simulink model "ELECTRIC_RC_AIRCRAFT_backup_2"  (R2025b)
settings: Solver=VariableStepAuto  StartTime=0.0  StopTime=10000  RelTol=1e-3
values from neighbouring files (symbols this model uses):
  g = 9.81    [ELECTRIC_RC_AIRCRAFT.m]
  m = 1.83    [ELECTRIC_RC_AIRCRAFT.m]
libraries: aerolibadyn x1, aerolibatmos2 x1, aerolibasang x1, aerolibbdyn x1, aerolibactuator x1, slpidlib x1, aerolibpropulsion2 x1
settings Model: PacingRate=10  Creator=papar  LastModifiedBy=papar

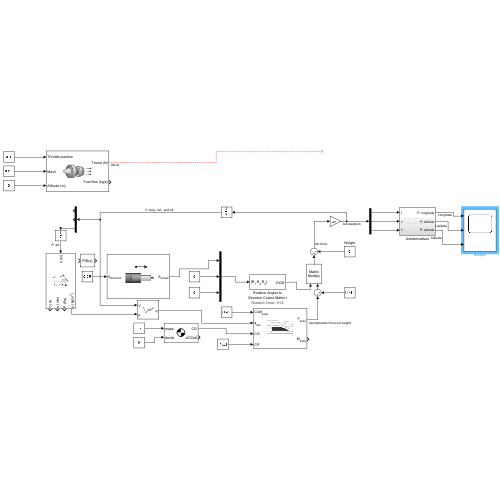
[thumbnail: Simulink's stored preview of the top-level diagram]
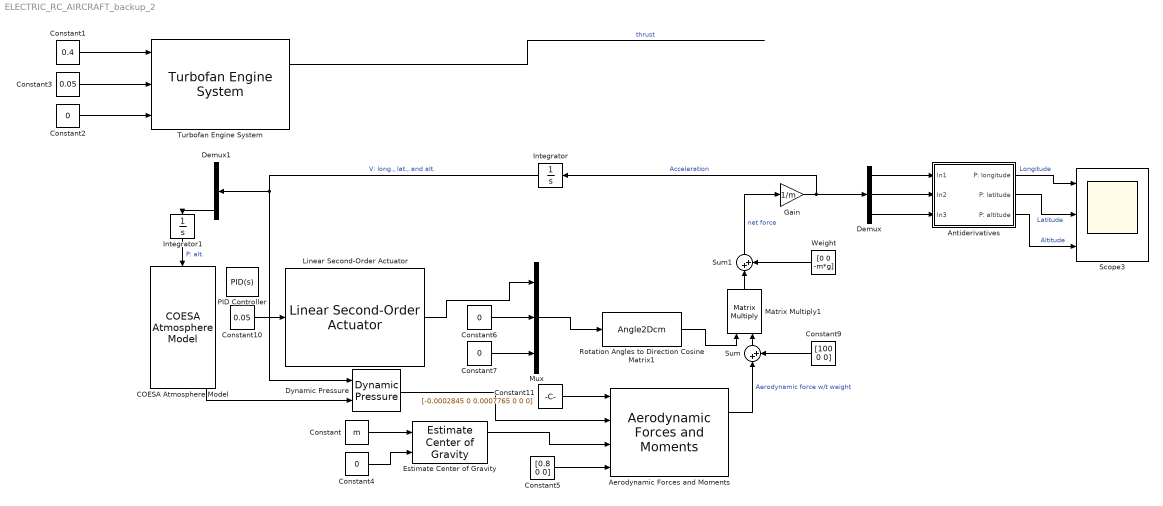
== system ELECTRIC_RC_AIRCRAFT_backup_2 ==
  "Aerodynamic Forces and Moments " : aerolibadyn/Aerodynamic Forces and Moments   inputAxes=Body  outputForceAxes=Body  outputMomentAxes=Body  S=1.67  b=3.66  cbar=2.13
  Antiderivatives : Subsystem
  COESA Atmosphere Model : aerolibatmos2/COESA Atmosphere Model  units=Metric (MKS)  spec=1976 COESA-extended U.S. Standard Atmosphere  model=Profile  profile_var=High temperature  profile_percent=1%  profile_alt=5 km (16404 ft)  envelope_var=High temperature  envelope_percent=1%  action=Warning
  Constant : Constant  Value=m
  Constant1 : Constant  Value=0.4
  Constant10 : Constant  Value=0.05
  Constant11 : Constant  Value=[-0.0002845 0 0.0007765 0 0 0]
  Constant{2,4,6..7} (4 alike) : Constant  Value=0
  Constant3 : Constant  Value=0.05
  Constant5 : Constant  Value=[0.8 0 0]
  Constant9 : Constant  Value=[100 0 0]
  Demux : Demux  Outputs=3
  Demux1 : Demux  Outputs=3
  Dynamic Pressure : aerolibasang/Dynamic Pressure
  Estimate Center of Gravity : aerolibbdyn/Estimate Center of Gravity  fmass=m  emass=m  fcg=[0 0 0]'  ecg=[0 0 0]'
  Gain : Gain  Gain=1/m
  Integrator : Integrator
  Integrator1 : Integrator
  Linear Second-Order Actuator : aerolibactuator/Linear Second-Order Actuator  wn_fin=8  z_fin=0.7  fin_act_0=0  fin_act_vel=0
  Matrix Multiply1 : Product  Multiplication=Matrix(*)
  Mux : Mux  Inputs=3
  PID Controller : slpidlib/PID Controller  Controller=PID  Form=Parallel  TimeDomain=Continuous-time  UseExternalTs=off  SampleTime=-1  IntegratorMethod=Forward Euler  FilterMethod=Forward Euler  ControllerParametersSource=internal  P=1  I=1  UseKiTs=off  D=0  UseExternalDerivativeSource=off  N=100  UseFilter=on  TunerSelectOption=Transfer Function Based (PID Tuner App)  InitialConditionSource=internal  InitialConditionForIntegrator=0  InitialConditionForFilter=0  DifferentiatorICPrevScaledInput=0  ExternalReset=none  TrackingMode=off  Kt=1  LimitOutput=off  SatLimitsSource=internal  UpperSaturationLimit=inf  LowerSaturationLimit=-inf  LinearizeAsGain=on  AntiWindupMode=none  Kb=1  LimitIntegrator=off  UpperIntegratorSaturationLimit=inf  LowerIntegratorSaturationLimit=-inf  POutMin=[]  POutMax=[]  IOutMin=[]  IOutMax=[]  DOutMin=[]  DOutMax=[]  NOutMin=[]  NOutMax=[]  SumOutMin=[]  SumOutMax=[]  SaturationOutMin=[]  SaturationOutMax=[]  PParamMin=[]  PParamMax=[]  IParamMin=[]  IParamMax=[]  DParamMin=[]  DParamMax=[]  NParamMin=[]  NParamMax=[]  KbParamMin=[]  KbParamMax=[]  KtParamMin=[]  KtParamMax=[]  KbOutMin=[]  KbOutMax=[]  KtOutMin=[]  KtOutMax=[]  IntegratorOutMin=[]  IntegratorOutMax=[]  FilterOutMin=[]  FilterOutMax=[]  SumI1OutMin=[]  SumI1OutMax=[]  SumI2OutMin=[]  SumI2OutMax=[]  SumI3OutMin=[]  SumI3OutMax=[]  SumI4OutMin=[]  SumI4OutMax=[]  SumDOutMin=[]  SumDOutMax=[]  DifferentiatorOutMin=[]  DifferentiatorOutMax=[]  FilterDiffOutCoefMin=[]  FilterDiffOutCoefMax=[]  ReciprocalOutMin=[]  ReciprocalOutMax=[]  SumDenOutMin=[]  SumDenOutMax=[]  SumNumOutMin=[]  SumNumOutMax=[]  DivideOutMin=[]  DivideOutMax=[]  UdiffTsProdOutMin=[]  UdiffTsProdOutMax=[]  NTsProdOutMin=[]  NTsProdOutMax=[]  UintegralTsProdOutMin=[]  UintegralTsProdOutMax=[]  UngainTsProdOutMin=[]  UngainTsProdOutMax=[]  ClampingZeroOutDataTypeStr=Inherit: Inherit via back propagation  ClampingZeroOutMin=[]  ClampingZeroOutMax=[]  FilterDenConstantOutDataTypeStr=Inherit: Inherit via back propagation  FilterDenConstantOutMin=[]  FilterDenConstantOutMax=[]  PCopyOutDataTypeStr=Inherit: Inherit via back propagation  PCopyOutMin=[]  PCopyOutMax=[]  NCopyOutDataTypeStr=Inherit: Inherit via back propagation  NCopyOutMin=[]  NCopyOutMax=[]  IntegratorContinuousStateAttributes=''  IntegratorStateMustResolveToSignalObject=off  IntegratorRTWStateStorageClass=Auto  FilterContinuousStateAttributes=''  FilterStateMustResolveToSignalObject=off  FilterRTWStateStorageClass=Auto  ParallelPVariant=InternalParameters  IdealPVariant=Disabled  IVariant=InternalParameters  DVariant=InternalParameters  IntegratorVariant=Continuous  SatVariant=Disabled  AWVariant=Passthrough  PCopyVariant=Disabled  TRVariant=Disabled  FdbkBlocksVariant=Forward  IdealPFdbkVariant=Disabled  SatFdbkVariant=Disabled  DerivativeFilterVariant=ContFilter  NVariant=InternalParameters  NCopyVariant=Disabled  FilterICVariant=InternalICsFilter  IntegratorICVariant=InternalICs  ExternalResetVariant=Disabled  TRSumVariant=Passthrough  SumFdbkVariant=Disabled  SumVariant=Sum_PID  TsampFilterVariant=InternalTs  TsampNgainVariant=Passthrough  TsampIntegralVariant=Disabled_SignalSpec  ExternalSaturationOutDataTypeStr=Inherit: Same as second input  DerivativeSourceVariant=ErrorSignal  PreIntVariant=InternalPreInt
  Rotation Angles to Direction Cosine Matrix1 : Angle2Dcm  rotationOrder=XYZ
      settings: AttributesFormatString=Rotation Order: %<rotationOrder>
  Scope3 : Scope  NumInputPorts=3
      settings: ActiveDisplayString=3  ActiveDisplayYMinimum=-396534.97594564385  ActiveDisplayYMaximum=190294.17453192952  DataLoggingVariableName=ScopeData2
  Sum : Sum  Inputs=|++
  Sum1 : Sum  Inputs=|++
  Turbofan Engine System : aerolibpropulsion2/Turbofan Engine System  units=Metric (MKS)  ic_source=Internal  IC=0  Fmax=20  tau=0.4  SFC=0  Nt=0.9
  Weight : Constant  Value=[0 0 -m*g]
  wires:
  Gain/1 -> Demux/1, Integrator/1  "Acceleration"
  Constant1/1 -> Turbofan Engine System/1
  Constant2/1 -> Turbofan Engine System/3
  Constant3/1 -> Turbofan Engine System/2
  Turbofan Engine System/1 -> ?  "thrust"
  Constant/1 -> Estimate Center of Gravity/1
  Constant4/1 -> Estimate Center of Gravity/2
  Constant11/1 -> "Aerodynamic Forces and Moments "/1
  Weight/1 -> Sum1/2
  Matrix Multiply1/1 -> Sum1/1
  Mux/1 -> Rotation Angles to Direction Cosine Matrix1/1
  Constant10/1 -> Linear Second-Order Actuator/1
  "Aerodynamic Forces and Moments "/1 -> Sum/1  "Aerodynamic force w/t weight"
  Rotation Angles to Direction Cosine Matrix1/1 -> Matrix Multiply1/1
  Sum/1 -> Matrix Multiply1/2
  Constant9/1 -> Sum/2
  Dynamic Pressure/1 -> "Aerodynamic Forces and Moments "/2
  COESA Atmosphere Model/4 -> Dynamic Pressure/2
  Sum1/1 -> Gain/1  "net force"
  Integrator/1 -> Demux1/1, Dynamic Pressure/1  "V: long., lat., and alt."
  Constant5/1 -> "Aerodynamic Forces and Moments "/4
  Estimate Center of Gravity/1 -> "Aerodynamic Forces and Moments "/3
  Linear Second-Order Actuator/1 -> Mux/1
  Constant6/1 -> Mux/2
  Demux/1 -> Antiderivatives/1(In1)
  Demux/2 -> Antiderivatives/2(In2)
  Demux/3 -> Antiderivatives/3(In3)
  Antiderivatives/1(P: longitude) -> Scope3/1  "Longitude"
  Antiderivatives/2(P: latitude) -> Scope3/2  "Latitude"
  Antiderivatives/3(P: altitude) -> Scope3/3  "Altitude"
  Demux1/3 -> Integrator1/1
  Integrator1/1 -> COESA Atmosphere Model/1  "P: alt."
  Constant7/1 -> Mux/3

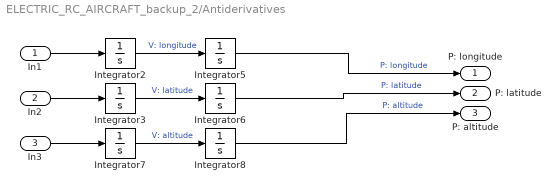
== system ELECTRIC_RC_AIRCRAFT_backup_2/Antiderivatives ==
  In1 : Inport
  In2 : Inport  Port=2
  In3 : Inport  Port=3
  Integrator{2..3,5..8} (6 alike) : Integrator
  P: longitude : Outport
  P: latitude : Outport  Port=2
  P: altitude : Outport  Port=3
  wires:
  Integrator7/1 -> Integrator8/1  "V: altitude"
  In2/1 -> Integrator3/1
  Integrator2/1 -> Integrator5/1  "V: longitude"
  Integrator8/1 -> P: altitude/1  "P: altitude"
  Integrator6/1 -> P: latitude/1  "P: latitude"
  Integrator3/1 -> Integrator6/1  "V: latitude"
  In3/1 -> Integrator7/1
  In1/1 -> Integrator2/1
  Integrator5/1 -> P: longitude/1  "P: longitude"
